simulink model "svm0127"  (R2023b)
settings: Solver=VariableStepAuto  StartTime=0.0  StopTime=10.0  RelTol=1e-3
InitFcn:
  | clear;
  | clc;
  | %Induction machine model
  | Rs=1.5313;
  | Rr=1.5313;
  | Rr1=Rr;
  | Rr=1*Rr;
  | M=0.21;
  | Ls=0.2194;
  | Lr=Ls;
  | Lls=0.0094;
  | Llr=Lls;
  | J=0.25;
  | P=4;
  | %B=0.0248;
  | Ts=Ls/Rs;
  | Tr=Lr/Rr1;
  | sigma=1-M*M/(Ls*Lr);
  | sigma_s=Lls/M;
  | sigma_r=Llr/M;
  | Kt=(2/3)*(P/2)*M/(1+sigma_r);
  | C=Lr*Ls-M*M;
  | G=17.4;
  | Imr_rated=6.439;
  | 
  | 
  | %Controller parameters
  | vsd_lim=13.015;
  | vsq_lim=26.613;
  | isq_lim=14.483*Kt*Imr_rated;
  | isd_lim=7.083;
  | Td=0.012; %d and q axis current controller
  | Kd=1.04;   %parameters
  | Kq=Kd/(Kt*Imr_rated);
  | Tc=.049725;     %Speed controller
  | Kc=18.204*Kt*Imr_rated;
  | 
  | Tfl=0.1432;     %Flux controller
  | Kfl=18/M;
  | %T1=25e-3;
  | %T2=3.5e-7;
  | 
  | %other parameters
  | Vdc=560;
undefined symbols (not defined in the file): magnitude
libraries: spsIGBTDiodeLib x6, spsVoltageMeasurementLib x3, spsDCVoltageSourceLib x2, spsCurrentMeasurementLib x1, spsAsynchronousMachineSIUnitsLib x1, simulink x1, spsThreePhaseVIMeasurementLib x1, sps_lib x1
settings Model: Creator=tyagi_av27qbo  LastModifiedBy=tyagi_av27qbo

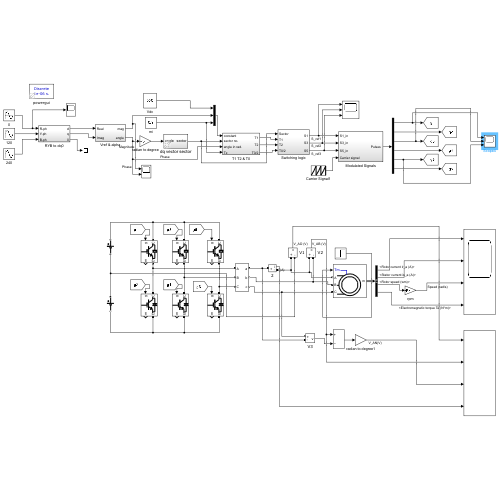
[thumbnail: Simulink's stored preview of the top-level diagram]
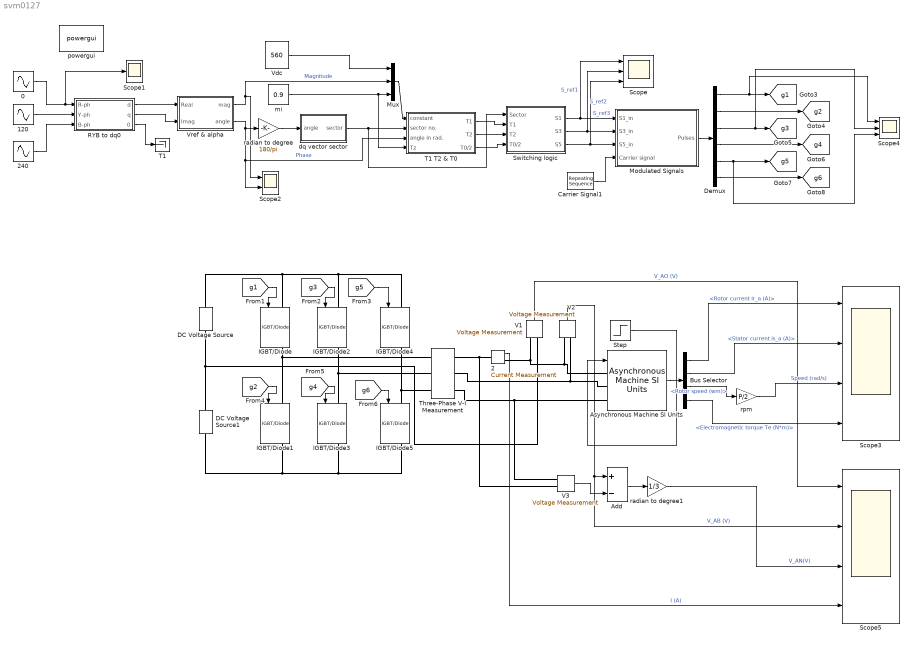
== system svm0127 ==
  0 : Sin  Amplitude=230*1.414  Frequency=2*pi*50  SampleTime=0
  120 : Sin  Amplitude=230*1.414  Frequency=2*pi*50  Phase=-(2*pi)/3  SampleTime=0
  2 : spsCurrentMeasurementLib/Current Measurement  PhasorSimulation=off  OutputType=Complex  PSBequivalent=0
  240 : Sin  Amplitude=230*1.414  Frequency=2*pi*50  Phase=(2*pi)/3  SampleTime=0
  Add : Sum  Inputs=+-
  Asynchronous Machine SI Units : spsAsynchronousMachineSIUnitsLib/Asynchronous Machine SI Units  RotorType=Squirrel-cage  PresetModel=No  MechanicalLoad=Torque Tm  ShowDetailedParameters=on  ReferenceFrame=Rotor  Units=SI  MeasurementBus=off  NominalParameters=[3000 400 50]  VoltageRatio=1  Stator=[Rs Lls]  Rotor=[Rr Llr]  Cage1=[0.4155 0.002066]  Cage2=[0.4168 0.0003495]  Lm=M  Mechanical=[J 0 2]  PolePairs=2  InitialConditions="[ 1,0   0,0,0   0,0,0 ]"  SimulateSaturation=off  Saturation=[14.03593122, 27.81365428, 53.79336849, 72.68890987, 97.98006896, 148.6815601, 215.7428561, 302.9841135, 428.7778367 ; 230, 322, 414, 460, 506, 552, 598, 644, 690]  LoadFlowParameters=1492000  TsPowergui=0  TsBlock=-1  IterativeModel=Trapezoidal non iterative  IterativeDiscreteModel=Trapezoidal non iterative  Pmec=0
  Bus Selector : BusSelector  OutputSignals=Rotor measurements.Rotor current ir_a (A),Stator measurements.Stator current is_a (A),Mechanical.Rotor speed (wm),Mechanical.Electromagnetic torque Te (N*m)
  Carrier Signal1 : simulink/Sources/Repeating Sequence  rep_seq_t=[0 .5 1]*(1/3000)  rep_seq_y=[0 .5 1]
  DC Voltage Source : spsDCVoltageSourceLib/DC Voltage Source  Amplitude=Vdc/2  Measurements=None
  DC Voltage Source1 : spsDCVoltageSourceLib/DC Voltage Source  Amplitude=Vdc/2  Measurements=None
  Demux : Demux  Outputs=6
  IGBT/Diode{,1..5} (6 alike) : spsIGBTDiodeLib/IGBT//Diode  Ron=1e-3  Rs=1e5  Cs=inf  Measurements=on
  Modulated Signals : Subsystem
  Mux : Mux  Inputs=3
  RYB to dq0 : Subsystem
  Scope : Scope  NumInputPorts=3
  Scope1 : Scope
  Scope2 : Scope  NumInputPorts=2
  Scope3 : Scope  NumInputPorts=4
  Scope4 : Scope  NumInputPorts=3
  Scope5 : Scope  NumInputPorts=4
  Step : Step  Time=2  After=23  SampleTime=0
  Switching logic : Subsystem
  T1 : Terminator
  T1 T2 & T0 : Subsystem
  Three-Phase V-I Measurement : spsThreePhaseVIMeasurementLib/Three-Phase V-I Measurement  VoltageMeasurement=phase-to-phase  SetLabelV=on  LabelV=Vabc  Vpu=off  VpuLL=off  CurrentMeasurement=yes  SetLabelI=on  LabelI=Iabc  Ipu=off  Pbase=100e6  Vbase=500e3  OutputType=Complex  PhasorSimulation=off  PSBequivalent=0
  V1 : spsVoltageMeasurementLib/Voltage Measurement  PhasorSimulation=off  OutputType=Complex  PSBequivalent=0
  V2 : spsVoltageMeasurementLib/Voltage Measurement  PhasorSimulation=off  OutputType=Complex  PSBequivalent=0
  V3 : spsVoltageMeasurementLib/Voltage Measurement  PhasorSimulation=off  OutputType=Complex  PSBequivalent=0
  Vdc : Constant  Value=560
  Vref & alpha : Subsystem
  dq vector sector : Subsystem  AncestorBlock=AC2DriveInternalModels/SVM generator/ab vector sector
  "mi " : Constant  Value=0.9
  powergui : sps_lib/powergui  Priority=1  SimulationMode=Discrete  SampleTime=1e-6  frequency=60  Iterations=50  frequencyindice=0  Pbase=100e6  ErrMax=1e-4  UnitsV=kV  UnitsW=MW  buscounter=0  FunctionMessages=off  echomessages=off  EnableUseOfTLC=off  CurrentSourceSwitches=off  DisableSnubberDevices=off  DisableRonSwitches=off  DisableVfSwitches=off  DisplayEquations=off  AutomaticDiscreteSolvers=off  SolverType=Tustin  Interpol=off  ExternalGateDelay=off  methode=off  Ts=0  x0status=blocks  SPID=off  SwTol=0  HookPort=off  NonlinearTolerance=1e-4  nMaxIteration=100  ContinueOnMaxIteration=off  RestoreLinks=warning  ResistiveCurrentMeasurement=off  Frange=[0:2:500]  Ylog=off  Xlog=on  ShowGrid=off  save=off  variable=ZData  structure=svm  ZoomFFT=off  StartTime=0.4  cycles=10  DisplayStyle=2  fundamental=50  FreqAxis=on  MaxFrequency=10000  frequencyindicesteady=1  RmsSteady=1  display=off
  radian to degree : Gain  Gain=180/pi
  radian to degree1 : Gain  Gain=1/3
  rpm : Gain  Gain=P/2  SaturateOnIntegerOverflow=on  OutDataTypeStr=Inherit: Same as input  ParamDataTypeStr=Inherit: Same as input
  tag scope: g1=global, g2=global, g3=global, g4=global, g5=global, g6=global
  wires:
  2/1 -> Scope5/4  "I (A)"
  V3/1 -> Add/2
  Bus Selector/4 -> Scope3/4  "<Electromagnetic torque Te (N*m)>"
  [g6] -> IGBT/Diode5/1
  [g2] -> IGBT/Diode1/1
  "mi "/1 -> Mux/3, T1 T2 & T0/4(Tz)
  Demux/5 -> Scope4/3, [g5]
  V2/1 -> Add/1, Scope5/2  "V_AB (V)"
  RYB to dq0/3(0) -> T1/1
  Switching logic/1(S1) -> Modulated Signals/1(S1_in), Scope/1  "S_ref1"
  radian to degree/1 -> dq vector sector/1(angle)
  [g1] -> IGBT/Diode/1
  [g3] -> IGBT/Diode2/1
  rpm/1 -> Scope3/3  "Speed (rad/s)"
  Asynchronous Machine SI Units/1 -> Bus Selector/1
  Bus Selector/1 -> Scope3/1  "<Rotor current ir_a (A)>"
  Bus Selector/3 -> rpm/1  "<Rotor speed (wm)>"
  Demux/2 -> [g2]
  Demux/3 -> Scope4/2, [g3]
  T1 T2 & T0/1(T1) -> Switching logic/2(T1)
  Demux/6 -> [g6]
  [g4] -> IGBT/Diode3/1
  [g5] -> IGBT/Diode4/1
  Modulated Signals/1("Pulses ") -> Demux/1
  Demux/4 -> [g4]
  120/1 -> RYB to dq0/2(Y-ph)
  Bus Selector/2 -> Scope3/2  "<Stator current is_a (A)>"
  Demux/1 -> Scope4/1, [g1]
  Vref & alpha/2(angle) -> radian to degree/1, Scope2/2, T1 T2 & T0/3(angle in rad.)  "Phase"
  RYB to dq0/1(d) -> Vref & alpha/1(Real)
  Vref & alpha/1(mag) -> Scope2/1, Mux/2  "Magnitude"
  dq vector sector/1(sector) -> T1 T2 & T0/2(sector no.), Switching logic/1(Sector)
  240/1 -> RYB to dq0/3(B-ph)
  RYB to dq0/2(q) -> Vref & alpha/2(Imag)
  Vdc/1 -> Mux/1
  0/1 -> Scope1/1, RYB to dq0/1(R-ph)
  Step/1 -> Asynchronous Machine SI Units/1
  T1 T2 & T0/2(T2) -> Switching logic/3(T2)
  V1/1 -> Scope5/1  "V_AO (V)"
  Mux/1 -> T1 T2 & T0/1(constant)
  Switching logic/2(S3) -> Scope/2, Modulated Signals/2(S3_in)  "S_ref2"
  Carrier Signal1/1 -> Modulated Signals/4("Carrier signal ")
  Add/1 -> radian to degree1/1
  Switching logic/3(S5) -> Scope/3, Modulated Signals/3(S5_in)  "S_ref3"
  T1 T2 & T0/3(T0/2) -> Switching logic/4(T0/2)
  radian to degree1/1 -> Scope5/3  "V_AN(V)"
  connections:
  DC Voltage Source/LConn1 -- DC Voltage Source1/RConn1 -- V1/LConn2
  2/LConn1 -- Three-Phase V-I Measurement/RConn1 -- V3/LConn2
  Three-Phase V-I Measurement/RConn2 -- Asynchronous Machine SI Units/LConn2 -- V2/LConn2
  IGBT/Diode1/LConn1 -- Three-Phase V-I Measurement/LConn1 -- IGBT/Diode/RConn1
  Asynchronous Machine SI Units/LConn3 -- Three-Phase V-I Measurement/RConn3 -- V3/LConn1
  IGBT/Diode3/LConn1 -- Three-Phase V-I Measurement/LConn2 -- IGBT/Diode2/RConn1
  IGBT/Diode3/RConn1 -- IGBT/Diode5/RConn1 -- IGBT/Diode1/RConn1 -- DC Voltage Source1/LConn1
  DC Voltage Source/RConn1 -- IGBT/Diode2/LConn1 -- IGBT/Diode4/LConn1 -- IGBT/Diode/LConn1
  IGBT/Diode4/RConn1 -- Three-Phase V-I Measurement/LConn3 -- IGBT/Diode5/LConn1
  Asynchronous Machine SI Units/LConn1 -- V1/LConn1 -- 2/RConn1 -- V2/LConn1

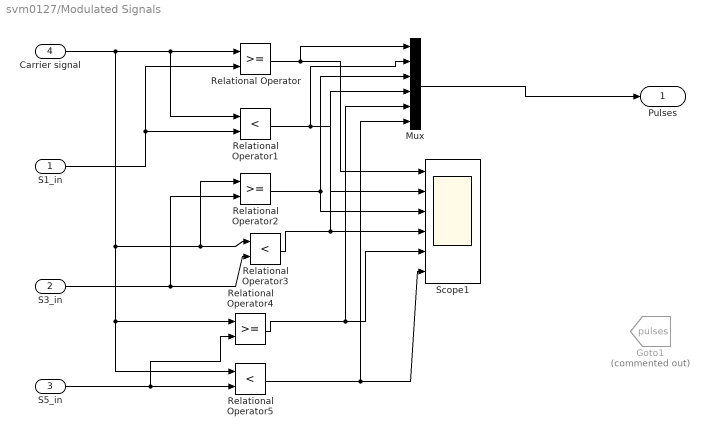
== system svm0127/Modulated Signals ==
  S1_in : Inport
  S3_in : Inport  Port=2
  S5_in : Inport  Port=3
  "Carrier signal " : Inport  Port=4
  Goto1 : Goto  Commented=on  GotoTag=pulses  TagVisibility=global
  Mux : Mux  Inputs=6
  Relational Operator : RelationalOperator  OutDataTypeStr=boolean  InputSameDT=off
  Relational Operator1 : RelationalOperator  Operator=<  OutDataTypeStr=boolean  InputSameDT=off
  Relational Operator2 : RelationalOperator  OutDataTypeStr=boolean  InputSameDT=off
  Relational Operator3 : RelationalOperator  Operator=<  OutDataTypeStr=boolean  InputSameDT=off
  Relational Operator4 : RelationalOperator  OutDataTypeStr=boolean  InputSameDT=off
  Relational Operator5 : RelationalOperator  Operator=<  OutDataTypeStr=boolean  InputSameDT=off
  Scope1 : Scope  NumInputPorts=6
  "Pulses " : Outport
  wires:
  "Carrier signal "/1 -> Relational Operator/1, Relational Operator1/1, Relational Operator2/1, Relational Operator3/1, Relational Operator4/1, Relational Operator5/1
  S1_in/1 -> Relational Operator/2, Relational Operator1/2
  S3_in/1 -> Relational Operator2/2, Relational Operator3/2
  Relational Operator/1 -> Scope1/1, Mux/1
  Relational Operator1/1 -> Scope1/2, Mux/2
  Relational Operator2/1 -> Scope1/3, Mux/3
  Relational Operator3/1 -> Scope1/4, Mux/4
  Relational Operator4/1 -> Scope1/5, Mux/5
  Relational Operator5/1 -> Scope1/6, Mux/6
  Mux/1 -> "Pulses "/1
  S5_in/1 -> Relational Operator4/2, Relational Operator5/2

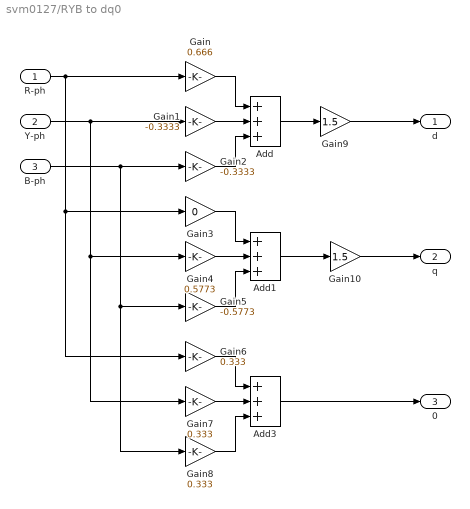
== system svm0127/RYB to dq0 ==
  R-ph : Inport
  Y-ph : Inport  Port=2
  B-ph : Inport  Port=3
  Add : Sum  Inputs=+++
  Add1 : Sum  Inputs=+++
  Add3 : Sum  Inputs=+++
  Gain : Gain  Gain=0.666
  Gain1 : Gain  Gain=-0.3333
  Gain10 : Gain  Gain=1.5
  Gain2 : Gain  Gain=-0.3333
  Gain3 : Gain  Gain=0
  Gain4 : Gain  Gain=0.5773
  Gain5 : Gain  Gain=-0.5773
  Gain6 : Gain  Gain=0.333
  Gain7 : Gain  Gain=0.333
  Gain8 : Gain  Gain=0.333
  Gain9 : Gain  Gain=1.5
  d : Outport
  q : Outport  Port=2
  0 : Outport  Port=3
  wires:
  B-ph/1 -> Gain5/1, Gain8/1, Gain2/1
  Gain/1 -> Add/1
  Gain1/1 -> Add/2
  Gain2/1 -> Add/3
  Add/1 -> Gain9/1
  Gain3/1 -> Add1/1
  Gain4/1 -> Add1/2
  Gain5/1 -> Add1/3
  Add1/1 -> Gain10/1
  Gain6/1 -> Add3/1
  Gain7/1 -> Add3/2
  Gain8/1 -> Add3/3
  Add3/1 -> 0/1
  R-ph/1 -> Gain/1, Gain3/1, Gain6/1
  Y-ph/1 -> Gain1/1, Gain7/1, Gain4/1
  Gain9/1 -> d/1
  Gain10/1 -> q/1

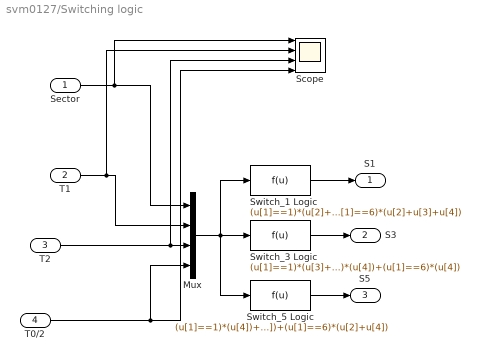
== system svm0127/Switching logic ==
  Sector : Inport
  T1 : Inport  Port=2
  T2 : Inport  Port=3
  T0/2 : Inport  Port=4
  Mux : Mux
  Scope : Scope  NumInputPorts=4
  Switch_1 Logic : Fcn  Expr=(u[1]==1)*(u[2]+u[3]+u[4])+(u[1]==2)*(u[2]+u[4])+(u[1]==3)*(u[4])+(u[1]==4)*(u[4])+(u[1]==5)*(u[3]+u[4])+(u[1]==6)*(u[2]+u[3]+u[4])
  Switch_3 Logic : Fcn  Expr=(u[1]==1)*(u[3]+u[4])+(u[1]==2)*(u[2]+u[3]+u[4])+(u[1]==3)*(u[2]+u[3]+u[4])+(u[1]==4)*(u[2]+u[4])+(u[1]==5)*(u[4])+(u[1]==6)*(u[4])
  Switch_5 Logic : Fcn  Expr=(u[1]==1)*(u[4])+(u[1]==2)*(u[4])+(u[1]==3)*(u[3]+u[4])+(u[1]==4)*(u[2]+u[3]+u[4])+(u[1]==5)*(u[2]+u[3]+u[4])+(u[1]==6)*(u[2]+u[4])
  S1 : Outport
  S3 : Outport  Port=2
  S5 : Outport  Port=3
  wires:
  Sector/1 -> Scope/1, Mux/1
  T1/1 -> Scope/2, Mux/2
  T2/1 -> Scope/3, Mux/3
  T0/2/1 -> Scope/4, Mux/4
  Mux/1 -> Switch_3 Logic/1, Switch_1 Logic/1, Switch_5 Logic/1
  Switch_1 Logic/1 -> S1/1
  Switch_3 Logic/1 -> S3/1
  Switch_5 Logic/1 -> S5/1

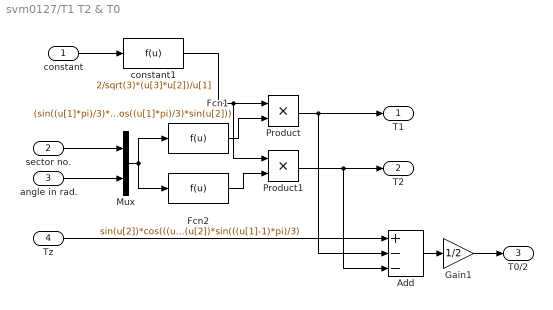
== system svm0127/T1 T2 & T0 ==
  constant : Inport
  sector no. : Inport  Port=2
  angle in rad. : Inport  Port=3
  Tz : Inport  Port=4
  Add : Sum  Inputs=+--
  Fcn1 : Fcn  Expr=(sin((u[1]*pi)/3)*cos(u[2]))-(cos((u[1]*pi)/3)*sin(u[2]))
  Fcn2 : Fcn  Expr=sin(u[2])*cos(((u[1]-1)*pi)/3)-cos(u[2])*sin(((u[1]-1)*pi)/3)
  Gain1 : Gain  Gain=1/2
  Mux : Mux  Inputs=2
  Product : Product  RndMeth=Zero
  Product1 : Product  RndMeth=Zero
  constant1 : Fcn  Expr=2/sqrt(3)*(u[3]*u[2])/u[1]
  T1 : Outport
  T2 : Outport  Port=2
  T0/2 : Outport  Port=3
  wires:
  Mux/1 -> Fcn1/1, Fcn2/1
  sector no./1 -> Mux/1
  angle in rad./1 -> Mux/2
  Fcn1/1 -> Product/2
  Fcn2/1 -> Product1/2
  Product/1 -> T1/1, Add/2
  Product1/1 -> T2/1, Add/3
  Tz/1 -> Add/1
  Add/1 -> Gain1/1
  Gain1/1 -> T0/2/1
  constant/1 -> constant1/1
  constant1/1 -> Product/1, Product1/1

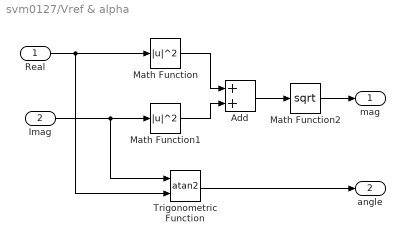
== system svm0127/Vref & alpha ==
  Real : Inport
  Imag : Inport  Port=2
  Add : Sum
  Math Function : Math  Operator=magnitude^2  SignedPower=on
  Math Function1 : Math  Operator=magnitude^2  SignedPower=on
  Math Function2 : Math  Operator=sqrt  SignedPower=on
  Trigonometric Function : Trigonometry  Operator=atan2
  mag : Outport
  angle : Outport  Port=2
  wires:
  Math Function/1 -> Add/1
  Math Function1/1 -> Add/2
  Add/1 -> Math Function2/1
  Math Function2/1 -> mag/1
  Real/1 -> Math Function/1, Trigonometric Function/2
  Imag/1 -> Math Function1/1, Trigonometric Function/1
  Trigonometric Function/1 -> angle/1

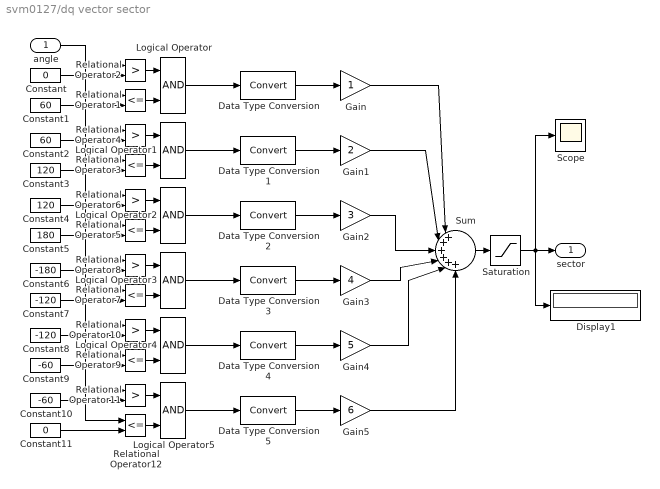
== system svm0127/dq vector sector ==
  angle : Inport
  Constant : Constant  Value=0
  Constant1 : Constant  Value=60
  Constant10 : Constant  Value=-60
  Constant11 : Constant  Value=0
  Constant2 : Constant  Value=60
  Constant3 : Constant  Value=120
  Constant4 : Constant  Value=120
  Constant5 : Constant  Value=180
  Constant6 : Constant  Value=-180
  Constant7 : Constant  Value=-120
  Constant8 : Constant  Value=-120
  Constant9 : Constant  Value=-60
  Data Type Conversion{,1..5} (6 alike) : DataTypeConversion
  Display1 : Display
  Gain : Gain  SaturateOnIntegerOverflow=on  OutDataTypeStr=Inherit: Same as input  ParamDataTypeStr=Inherit: Same as input
  Gain1 : Gain  Gain=2  SaturateOnIntegerOverflow=on  OutDataTypeStr=Inherit: Same as input  ParamDataTypeStr=Inherit: Same as input
  Gain2 : Gain  Gain=3  SaturateOnIntegerOverflow=on  OutDataTypeStr=Inherit: Same as input  ParamDataTypeStr=Inherit: Same as input
  Gain3 : Gain  Gain=4  SaturateOnIntegerOverflow=on  OutDataTypeStr=Inherit: Same as input  ParamDataTypeStr=Inherit: Same as input
  Gain4 : Gain  Gain=5  SaturateOnIntegerOverflow=on  OutDataTypeStr=Inherit: Same as input  ParamDataTypeStr=Inherit: Same as input
  Gain5 : Gain  Gain=6  SaturateOnIntegerOverflow=on  OutDataTypeStr=Inherit: Same as input  ParamDataTypeStr=Inherit: Same as input
  Logical Operator{,1..5} (6 alike) : Logic
  Relational Operator{1,3,5,7,9,12} (6 alike) : RelationalOperator  Operator=<=
  Relational Operator{2,4,6,8,10..11} (6 alike) : RelationalOperator  Operator=>
  Saturation : Saturate  UpperLimit=6  LowerLimit=1
  Scope : Scope
  Sum : Sum  Inputs=|++++++  InputSameDT=on  SaturateOnIntegerOverflow=on  OutDataTypeStr=Inherit: Same as first input
  sector : Outport
  wires:
  Data Type Conversion5/1 -> Gain5/1
  Data Type Conversion4/1 -> Gain4/1
  Data Type Conversion3/1 -> Gain3/1
  Data Type Conversion2/1 -> Gain2/1
  Data Type Conversion1/1 -> Gain1/1
  Data Type Conversion/1 -> Gain/1
  Relational Operator2/1 -> Logical Operator/1
  Relational Operator1/1 -> Logical Operator/2
  Logical Operator/1 -> Data Type Conversion/1
  angle/1 -> Relational Operator2/1, Relational Operator1/1, Relational Operator4/1, Relational Operator3/1, Relational Operator6/1, Relational Operator5/1, Relational Operator8/1, Relational Operator7/1, Relational Operator10/1, Relational Operator9/1, Relational Operator11/1, Relational Operator12/1
  Constant/1 -> Relational Operator2/2
  Constant1/1 -> Relational Operator1/2
  Relational Operator4/1 -> Logical Operator1/1
  Relational Operator3/1 -> Logical Operator1/2
  Logical Operator1/1 -> Data Type Conversion1/1
  Constant2/1 -> Relational Operator4/2
  Constant3/1 -> Relational Operator3/2
  Relational Operator6/1 -> Logical Operator2/1
  Relational Operator5/1 -> Logical Operator2/2
  Logical Operator2/1 -> Data Type Conversion2/1
  Constant4/1 -> Relational Operator6/2
  Constant5/1 -> Relational Operator5/2
  Relational Operator8/1 -> Logical Operator3/1
  Relational Operator7/1 -> Logical Operator3/2
  Logical Operator3/1 -> Data Type Conversion3/1
  Constant6/1 -> Relational Operator8/2
  Constant7/1 -> Relational Operator7/2
  Relational Operator10/1 -> Logical Operator4/1
  Relational Operator9/1 -> Logical Operator4/2
  Logical Operator4/1 -> Data Type Conversion4/1
  Constant8/1 -> Relational Operator10/2
  Constant9/1 -> Relational Operator9/2
  Relational Operator11/1 -> Logical Operator5/1
  Relational Operator12/1 -> Logical Operator5/2
  Logical Operator5/1 -> Data Type Conversion5/1
  Constant10/1 -> Relational Operator11/2
  Constant11/1 -> Relational Operator12/2
  Gain/1 -> Sum/1
  Gain1/1 -> Sum/2
  Gain2/1 -> Sum/3
  Gain3/1 -> Sum/4
  Gain4/1 -> Sum/5
  Gain5/1 -> Sum/6
  Sum/1 -> Saturation/1
  Saturation/1 -> Display1/1, Scope/1, sector/1
